simulink model "wr_model"  (R2018b)
settings: Solver=VariableStepAuto  StartTime=0.0  StopTime=20  FixedStep=1  MaxStep=10.0  RelTol=1e-3
undefined symbols (not defined in the file): water, wr
libraries: simulink x4
settings Model: Creator=martin  LastModifiedBy=felix
settings DataIOCC: OutputSaveName=State

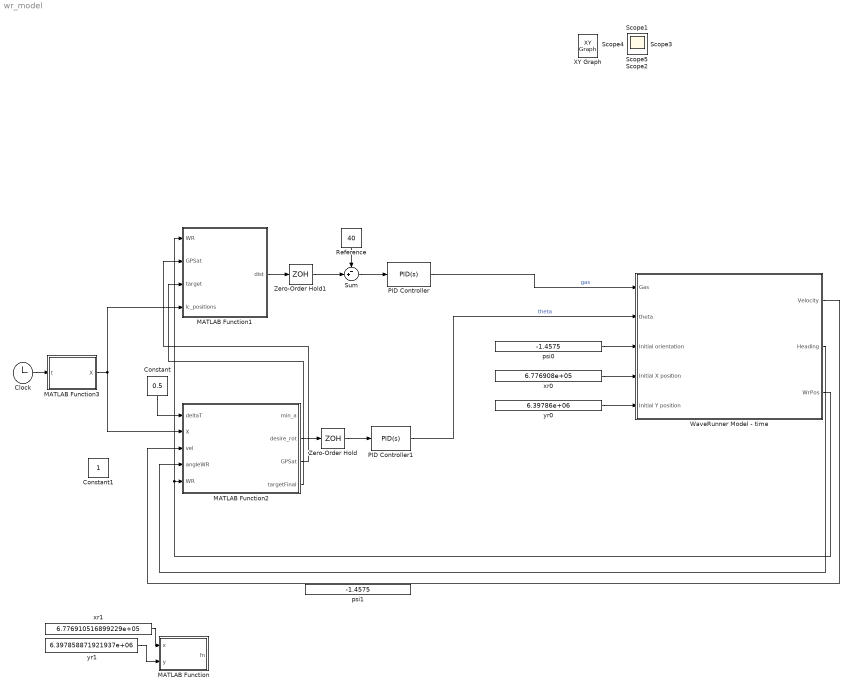
== system wr_model ==
  Clock : Clock
      settings: Decimation=1000
  Constant : Constant  Value=0.5
  Constant1 : Constant
  MATLAB Function : MATLAB Function  TreatAsAtomicUnit=on
  MATLAB Function1 : MATLAB Function  TreatAsAtomicUnit=on
  MATLAB Function2 : MATLAB Function  TreatAsAtomicUnit=on
  MATLAB Function3 : MATLAB Function  TreatAsAtomicUnit=on
  PID Controller : simulink/Continuous/PID Controller  Controller=PID  Form=Parallel  TimeDomain=Continuous-time  SampleTime=-1  IntegratorMethod=Forward Euler  FilterMethod=Forward Euler  ControllerParametersSource=internal  P=1  I=0  D=1  UseFilter=on  N=100  TunerSelectOption=Transfer Function Based (PID Tuner App)  InitialConditionSource=internal  InitialConditionForIntegrator=0  InitialConditionForFilter=0  DifferentiatorICPrevScaledInput=0  ExternalReset=none  TrackingMode=off  Kt=1  LimitOutput=on  UpperSaturationLimit=100  LowerSaturationLimit=0  LinearizeAsGain=off  AntiWindupMode=none  Kb=1  POutMin=[]  POutMax=[]  IOutMin=[]  IOutMax=[]  DOutMin=[]  DOutMax=[]  NOutMin=[]  NOutMax=[]  SumOutMin=[]  SumOutMax=[]  SaturationOutMin=[]  SaturationOutMax=[]  PParamMin=[]  PParamMax=[]  IParamMin=[]  IParamMax=[]  DParamMin=[]  DParamMax=[]  NParamMin=[]  NParamMax=[]  KbParamMin=[]  KbParamMax=[]  KtParamMin=[]  KtParamMax=[]  KbOutMin=[]  KbOutMax=[]  KtOutMin=[]  KtOutMax=[]  IntegratorOutMin=[]  IntegratorOutMax=[]  FilterOutMin=[]  FilterOutMax=[]  SumI1OutMin=[]  SumI1OutMax=[]  SumI2OutMin=[]  SumI2OutMax=[]  SumI3OutMin=[]  SumI3OutMax=[]  SumI4OutMin=[]  SumI4OutMax=[]  SumDOutMin=[]  SumDOutMax=[]  DifferentiatorOutMin=[]  DifferentiatorOutMax=[]  FilterDiffOutCoefMin=[]  FilterDiffOutCoefMax=[]  ReciprocalOutMin=[]  ReciprocalOutMax=[]  SumDenOutMin=[]  SumDenOutMax=[]  SumNumOutMin=[]  SumNumOutMax=[]  DivideOutMin=[]  DivideOutMax=[]  IntegratorContinuousStateAttributes=''  IntegratorStateMustResolveToSignalObject=off  IntegratorRTWStateStorageClass=Auto  FilterContinuousStateAttributes=''  FilterStateMustResolveToSignalObject=off  FilterRTWStateStorageClass=Auto  ParallelPVariant=InternalParameters  IdealPVariant=Disabled  IVariant=InternalParameters  DVariant=InternalParameters  IntegratorVariant=Continuous  SatVariant=Enabled  AWVariant=Passthrough  PCopyVariant=Disabled  TRVariant=Disabled  FdbkBlocksVariant=Forward  IdealPFdbkVariant=Disabled  SatFdbkVariant=Disabled  DerivativeFilterVariant=ContFilter  NVariant=InternalParameters  NCopyVariant=Disabled  FilterICVariant=InternalICsFilter  IntegratorICVariant=InternalICs  ExternalResetVariant=Disabled  TRSumVariant=Passthrough  SumFdbkVariant=Disabled  SumVariant=Sum_PID
  PID Controller1 : simulink/Continuous/PID Controller  Controller=PID  Form=Parallel  TimeDomain=Continuous-time  SampleTime=-1  IntegratorMethod=Forward Euler  FilterMethod=Forward Euler  ControllerParametersSource=internal  P=1  I=0  D=0  UseFilter=on  N=100  TunerSelectOption=Transfer Function Based (PID Tuner App)  InitialConditionSource=internal  InitialConditionForIntegrator=0  InitialConditionForFilter=0  DifferentiatorICPrevScaledInput=0  ExternalReset=none  TrackingMode=off  Kt=1  LimitOutput=on  UpperSaturationLimit=24*pi/180  LowerSaturationLimit=-24*pi/180  LinearizeAsGain=off  AntiWindupMode=none  Kb=1  POutMin=[]  POutMax=[]  IOutMin=[]  IOutMax=[]  DOutMin=[]  DOutMax=[]  NOutMin=[]  NOutMax=[]  SumOutMin=[]  SumOutMax=[]  SaturationOutMin=[]  SaturationOutMax=[]  PParamMin=[]  PParamMax=[]  IParamMin=[]  IParamMax=[]  DParamMin=[]  DParamMax=[]  NParamMin=[]  NParamMax=[]  KbParamMin=[]  KbParamMax=[]  KtParamMin=[]  KtParamMax=[]  KbOutMin=[]  KbOutMax=[]  KtOutMin=[]  KtOutMax=[]  IntegratorOutMin=[]  IntegratorOutMax=[]  FilterOutMin=[]  FilterOutMax=[]  SumI1OutMin=[]  SumI1OutMax=[]  SumI2OutMin=[]  SumI2OutMax=[]  SumI3OutMin=[]  SumI3OutMax=[]  SumI4OutMin=[]  SumI4OutMax=[]  SumDOutMin=[]  SumDOutMax=[]  DifferentiatorOutMin=[]  DifferentiatorOutMax=[]  FilterDiffOutCoefMin=[]  FilterDiffOutCoefMax=[]  ReciprocalOutMin=[]  ReciprocalOutMax=[]  SumDenOutMin=[]  SumDenOutMax=[]  SumNumOutMin=[]  SumNumOutMax=[]  DivideOutMin=[]  DivideOutMax=[]  IntegratorContinuousStateAttributes=''  IntegratorStateMustResolveToSignalObject=off  IntegratorRTWStateStorageClass=Auto  FilterContinuousStateAttributes=''  FilterStateMustResolveToSignalObject=off  FilterRTWStateStorageClass=Auto  ParallelPVariant=InternalParameters  IdealPVariant=Disabled  IVariant=InternalParameters  DVariant=InternalParameters  IntegratorVariant=Continuous  SatVariant=Enabled  AWVariant=Passthrough  PCopyVariant=Disabled  TRVariant=Disabled  FdbkBlocksVariant=Forward  IdealPFdbkVariant=Disabled  SatFdbkVariant=Disabled  DerivativeFilterVariant=ContFilter  NVariant=InternalParameters  NCopyVariant=Disabled  FilterICVariant=InternalICsFilter  IntegratorICVariant=InternalICs  ExternalResetVariant=Disabled  TRSumVariant=Passthrough  SumFdbkVariant=Disabled  SumVariant=Sum_PID
  Reference : Constant  Value=40
  Sum : Sum  Inputs=-+|
  WaveRunner Model - time : Subsystem
  Zero-Order Hold : ZeroOrderHold
  Zero-Order Hold1 : ZeroOrderHold
  psi0 : Constant  Value=-1.4575
  psi1 : Constant  Value=-1.4575
  xr0 : Constant  Value=6.776908e+05
  xr1 : Constant  Value=6.776910516899229e+05
  yr0 : Constant  Value=6.39786e+06
  yr1 : Constant  Value=6.397858871921937e+06
  Scope{,1..5} (6 alike) : Scope
  XY Graph : simulink/Sinks/XY Graph  IOType=viewer  xmin=-1  xmax=1  ymin=-1  ymax=1  st=-1
  wires:
  Clock/1 -> MATLAB Function3/1(t)
  MATLAB Function3/1(X) -> MATLAB Function1/4(lc_positions), MATLAB Function2/2(X)
  Constant/1 -> MATLAB Function2/1(deltaT)
  Reference/1 -> Sum/1
  MATLAB Function1/1(dist) -> Zero-Order Hold1/1
  psi0/1 -> WaveRunner Model - time/3(Initial orientation)
  xr0/1 -> WaveRunner Model - time/4(Initial X position)
  yr0/1 -> WaveRunner Model - time/5(Initial Y position)
  MATLAB Function2/3(GPSat) -> MATLAB Function1/2(GPSat)
  MATLAB Function2/4(targetFinal) -> MATLAB Function1/3(target)
  xr1/1 -> MATLAB Function/1(x)
  yr1/1 -> MATLAB Function/2(y)
  WaveRunner Model - time/3(WrPos) -> MATLAB Function1/1(WR), MATLAB Function2/5(WR)
  Zero-Order Hold/1 -> PID Controller1/1
  MATLAB Function2/2(desire_rot) -> Zero-Order Hold/1
  Zero-Order Hold1/1 -> Sum/2
  WaveRunner Model - time/2(Heading) -> MATLAB Function2/4(angleWR)
  WaveRunner Model - time/1(Velocity) -> MATLAB Function2/3(vel)
  Sum/1 -> PID Controller/1
  PID Controller/1 -> WaveRunner Model - time/1(Gas)  "gas"
  PID Controller1/1 -> WaveRunner Model - time/2(theta)  "theta"

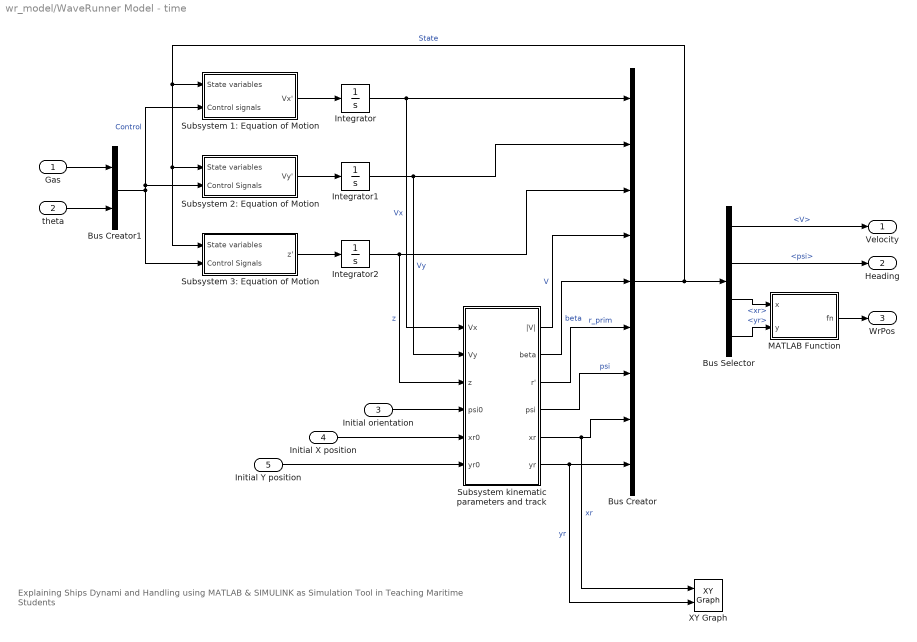
== system wr_model/WaveRunner Model - time ==
  note: Explaining Ships Dynami and Handling using MATLAB & SIMULINK as Simulation Tool in Teaching Maritime Students
  Gas : Inport
  theta : Inport  Port=2
  Initial orientation : Inport  Port=3
  Initial X position : Inport  Port=4
  Initial Y position : Inport  Port=5
  Bus Creator : BusCreator  Inputs=9
  Bus Creator1 : BusCreator  Inputs=2
  Bus Selector : BusSelector  OutputSignals=V,psi,xr,yr
  Integrator : Integrator
  Integrator1 : Integrator
  Integrator2 : Integrator
  MATLAB Function : MATLAB Function  TreatAsAtomicUnit=on
  Subsystem 1: Equation of Motion : Subsystem
  Subsystem 2: Equation of Motion : Subsystem
  Subsystem 3: Equation of Motion : Subsystem
  Subsystem kinematic parameters and track : Subsystem
  XY Graph : simulink/Sinks/XY Graph  xmin=6.65510516899229e+05  xmax=6.796910516899229e+05  ymin=6.308058871921937e+06  ymax=6.417858871921937e+06  st=-1
  Velocity : Outport
  Heading : Outport  Port=2
  WrPos : Outport  Port=3
  wires:
  Initial X position/1 -> Subsystem kinematic parameters and track/5(xr0)
  Subsystem 2: Equation of Motion/1(Vy') -> Integrator1/1
  Bus Creator/1 -> Subsystem 3: Equation of Motion/1(State variables), Subsystem 2: Equation of Motion/1(State variables), Subsystem 1: Equation of Motion/1(State variables), Bus Selector/1  "State"
  Integrator2/1 -> Subsystem kinematic parameters and track/3(z), Bus Creator/3  "z"
  Initial orientation/1 -> Subsystem kinematic parameters and track/4(psi0)
  Subsystem kinematic parameters and track/3(r') -> Bus Creator/6  "r_prim"
  Subsystem 1: Equation of Motion/1(Vx') -> Integrator/1
  Subsystem kinematic parameters and track/5(xr) -> XY Graph/1, Bus Creator/8  "xr"
  Subsystem kinematic parameters and track/6(yr) -> XY Graph/2, Bus Creator/9  "yr"
  Subsystem kinematic parameters and track/2(beta) -> Bus Creator/5  "beta"
  Bus Creator1/1 -> Subsystem 1: Equation of Motion/2(Control signals), Subsystem 2: Equation of Motion/2(Control Signals), Subsystem 3: Equation of Motion/2(Control Signals)  "Control"
  Subsystem kinematic parameters and track/4(psi) -> Bus Creator/7  "psi"
  Gas/1 -> Bus Creator1/1
  Integrator1/1 -> Subsystem kinematic parameters and track/2(Vy), Bus Creator/2  "Vy"
  Initial Y position/1 -> Subsystem kinematic parameters and track/6(yr0)
  Subsystem 3: Equation of Motion/1(z') -> Integrator2/1
  Subsystem kinematic parameters and track/1(|V|) -> Bus Creator/4  "V"
  Integrator/1 -> Bus Creator/1, Subsystem kinematic parameters and track/1(Vx)  "Vx"
  Bus Selector/2 -> Heading/1  "<psi>"
  Bus Selector/1 -> Velocity/1  "<V>"
  MATLAB Function/1(fn) -> WrPos/1
  theta/1 -> Bus Creator1/2
  Bus Selector/3 -> MATLAB Function/1(x)  "<xr>"
  Bus Selector/4 -> MATLAB Function/2(y)  "<yr>"

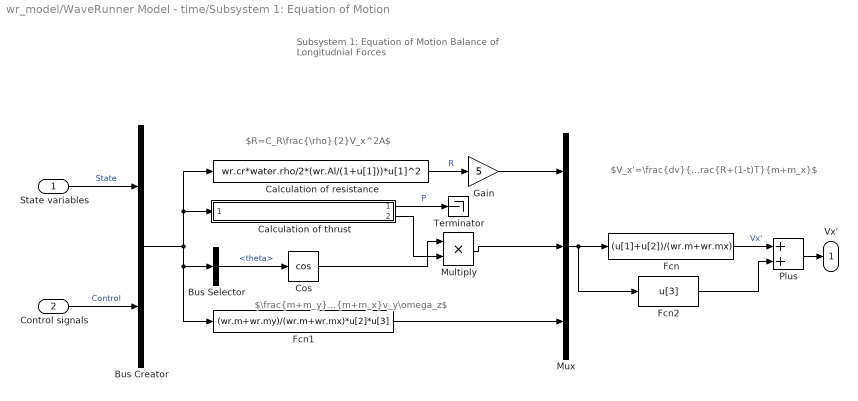
== system wr_model/WaveRunner Model - time/Subsystem 1: Equation of Motion ==
  note: $\frac{m+m_y}{m+m_x}v_y\omega_z$
  note: Subsystem 1: Equation of Motion
      | Balance of Longitudnial Forces
  note: $V_x'=\frac{dv}{dt}=\frac{R+(1-t)T}{m+m_x}$
  note: $R=C_R\frac{\rho}{2}V_x^2A$
  State variables : Inport
  Control signals : Inport  Port=2
  Bus Creator : BusCreator  Inputs=2  OutDataTypeStr=Bus: slBus1
  Bus Selector : BusSelector  OutputSignals=Control.theta
  Calculation of resistance : Fcn  Expr=wr.cr*water.rho/2*(wr.Al/(1+u[1]))*u[1]^2
  Calculation of thrust : ModelReference  ModelNameDialog=calculation_of_thrust  SimulationMode=Normal  ModelReferenceVersion=1.28
  Cos : Trigonometry  Operator=cos
  Fcn : Fcn  Expr=(u[1]+u[2])/(wr.m+wr.mx)
  Fcn1 : Fcn  Expr=(wr.m+wr.my)/(wr.m+wr.mx)*u[2]*u[3]
  Fcn2 : Fcn  Expr=u[3]
  Gain : Gain  Gain=5
  Multiply : Product
  Mux : Mux  Inputs=3
  Plus : Sum
  Terminator : Terminator
  Vx' : Outport
  wires:
  Mux/1 -> Fcn2/1, Fcn/1
  Calculation of resistance/1 -> Gain/1  "R"
  Control signals/1 -> Bus Creator/2  "Control"
  State variables/1 -> Bus Creator/1  "State"
  Plus/1 -> Vx'/1
  Bus Selector/1 -> Cos/1  "<theta>"
  Cos/1 -> Multiply/1
  Fcn1/1 -> Mux/3
  Bus Creator/1 -> Fcn1/1, Bus Selector/1, Calculation of resistance/1, Calculation of thrust/1
  Fcn/1 -> Plus/1  "Vx'"
  Fcn2/1 -> Plus/2
  Multiply/1 -> Mux/2
  Calculation of thrust/1 -> Terminator/1  "P"
  Gain/1 -> Mux/1
  Calculation of thrust/2 -> Multiply/2

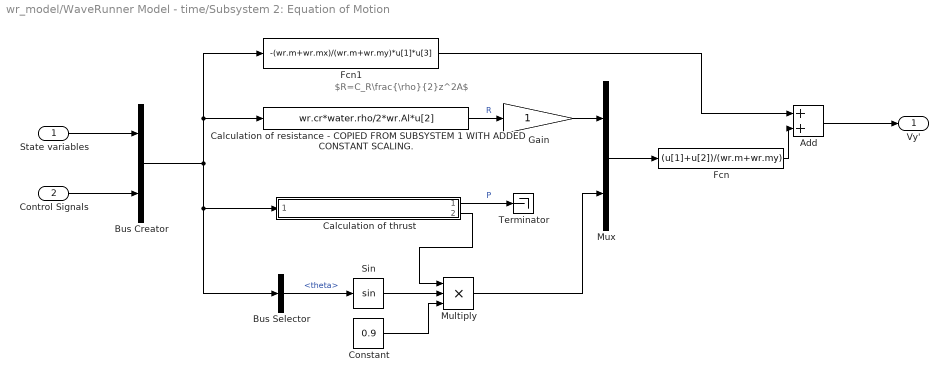
== system wr_model/WaveRunner Model - time/Subsystem 2: Equation of Motion ==
  note: $R=C_R\frac{\rho}{2}z^2A$
  State variables : Inport
  Control Signals : Inport  Port=2
  Add : Sum
  Bus Creator : BusCreator  Inputs=2
  Bus Selector : BusSelector  OutputSignals=Control.theta
  Calculation of resistance - COPIED FROM SUBSYSTEM 1 WITH ADDED CONSTANT SCALING. : Fcn  Expr=wr.cr*water.rho/2*wr.Al*u[2]
  Calculation of thrust : ModelReference  ModelNameDialog=calculation_of_thrust  SimulationMode=Normal  ModelReferenceVersion=1.28
  Constant : Constant  Value=0.9
  Fcn : Fcn  Expr=(u[1]+u[2])/(wr.m+wr.my)
  Fcn1 : Fcn  Expr=-(wr.m+wr.mx)/(wr.m+wr.my)*u[1]*u[3]
  Gain : Gain
  Multiply : Product  Inputs=3
  Mux : Mux  Inputs=2
  Sin : Trigonometry
  Terminator : Terminator
  Vy' : Outport
  wires:
  State variables/1 -> Bus Creator/1
  Control Signals/1 -> Bus Creator/2
  Calculation of resistance - COPIED FROM SUBSYSTEM 1 WITH ADDED CONSTANT SCALING./1 -> Gain/1  "R"
  Sin/1 -> Multiply/2
  Bus Selector/1 -> Sin/1  "<theta>"
  Constant/1 -> Multiply/3
  Bus Creator/1 -> Bus Selector/1, Calculation of thrust/1, Fcn1/1, Calculation of resistance - COPIED FROM SUBSYSTEM 1 WITH ADDED CONSTANT SCALING./1
  Mux/1 -> Fcn/1
  Gain/1 -> Mux/1
  Multiply/1 -> Mux/2
  Fcn/1 -> Add/2
  Fcn1/1 -> Add/1
  Add/1 -> Vy'/1
  Calculation of thrust/1 -> Terminator/1  "P"
  Calculation of thrust/2 -> Multiply/1

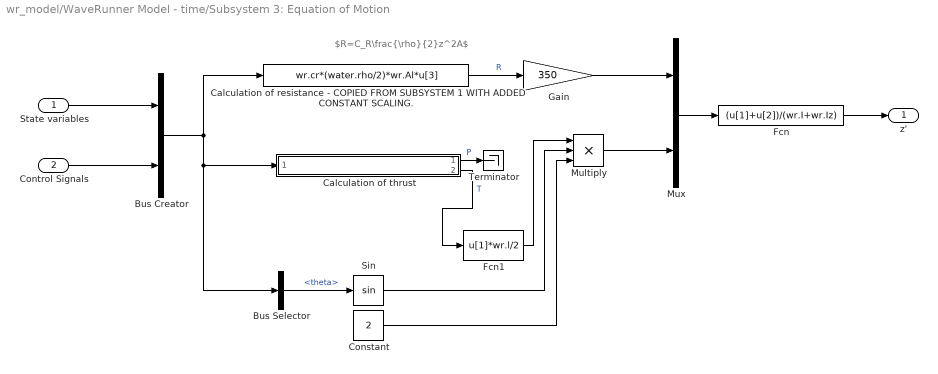
== system wr_model/WaveRunner Model - time/Subsystem 3: Equation of Motion ==
  note: $R=C_R\frac{\rho}{2}z^2A$
  State variables : Inport
  Control Signals : Inport  Port=2
  Bus Creator : BusCreator  Inputs=2
  Bus Selector : BusSelector  OutputSignals=Control.theta
  Calculation of resistance - COPIED FROM SUBSYSTEM 1 WITH ADDED CONSTANT SCALING. : Fcn  Expr=wr.cr*(water.rho/2)*wr.Al*u[3]
  Calculation of thrust : ModelReference  ModelNameDialog=calculation_of_thrust  SimulationMode=Normal  ModelReferenceVersion=1.28
  Constant : Constant  Value=2
  Fcn : Fcn  Expr=(u[1]+u[2])/(wr.I+wr.Iz)
  Fcn1 : Fcn  Expr=u[1]*wr.l/2
  Gain : Gain  Gain=350
  Multiply : Product  Inputs=3
  Mux : Mux  Inputs=2
  Sin : Trigonometry
  Terminator : Terminator
  z' : Outport
  wires:
  Control Signals/1 -> Bus Creator/2
  State variables/1 -> Bus Creator/1
  Sin/1 -> Multiply/2
  Bus Selector/1 -> Sin/1  "<theta>"
  Bus Creator/1 -> Calculation of resistance - COPIED FROM SUBSYSTEM 1 WITH ADDED CONSTANT SCALING./1, Bus Selector/1, Calculation of thrust/1
  Calculation of resistance - COPIED FROM SUBSYSTEM 1 WITH ADDED CONSTANT SCALING./1 -> Gain/1  "R"
  Multiply/1 -> Mux/2
  Fcn/1 -> z'/1
  Mux/1 -> Fcn/1
  Gain/1 -> Mux/1
  Fcn1/1 -> Multiply/1
  Calculation of thrust/2 -> Fcn1/1  "T"
  Calculation of thrust/1 -> Terminator/1  "P"
  Constant/1 -> Multiply/3

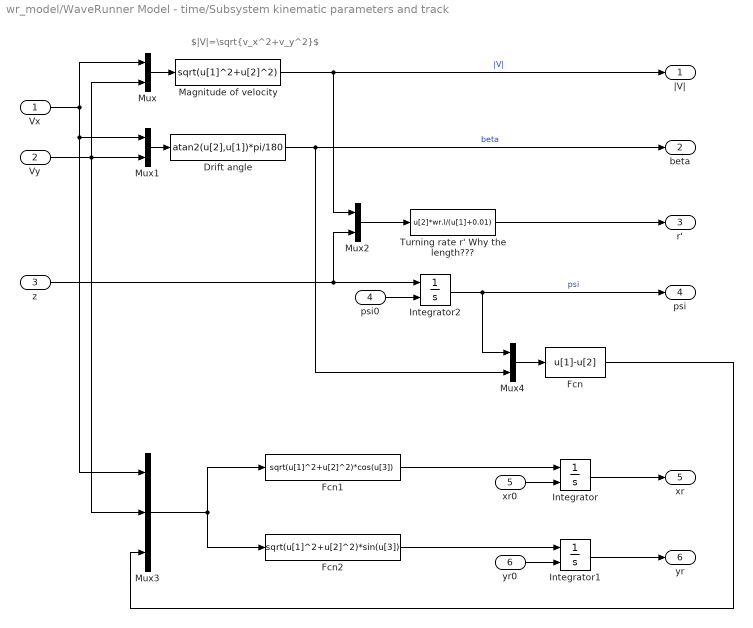
== system wr_model/WaveRunner Model - time/Subsystem kinematic parameters and track ==
  note: $|V|=\sqrt{v_x^2+v_y^2}$
  Vx : Inport
  Vy : Inport  Port=2
  z : Inport  Port=3
  psi0 : Inport  Port=4
  xr0 : Inport  Port=5
  yr0 : Inport  Port=6
  Drift angle : Fcn  Expr=atan2(u[2],u[1])*pi/180
  Fcn : Fcn  Expr=u[1]-u[2]
  Fcn1 : Fcn  Expr=sqrt(u[1]^2+u[2]^2)*cos(u[3])
  Fcn2 : Fcn  Expr=sqrt(u[1]^2+u[2]^2)*sin(u[3])
  Integrator : Integrator  InitialConditionSource=external
  Integrator1 : Integrator  InitialConditionSource=external
  Integrator2 : Integrator  InitialConditionSource=external
  Magnitude of velocity : Fcn  Expr=sqrt(u[1]^2+u[2]^2)
  Mux{,1..2,4} (4 alike) : Mux  Inputs=2
  Mux3 : Mux  Inputs=3
  Turning rate r' Why the length??? : Fcn  Expr=u[2]*wr.l/(u[1]+0.01)
  |V| : Outport
  beta : Outport  Port=2
  r' : Outport  Port=3
  psi : Outport  Port=4
  xr : Outport  Port=5
  yr : Outport  Port=6
  wires:
  Mux/1 -> Magnitude of velocity/1
  Magnitude of velocity/1 -> Mux2/1, |V|/1  "|V|"
  Vx/1 -> Mux/1, Mux3/1, Mux1/1
  Vy/1 -> Mux/2, Mux3/2, Mux1/2
  Integrator1/1 -> yr/1
  Integrator/1 -> xr/1
  Integrator2/1 -> Mux4/1, psi/1  "psi"
  psi0/1 -> Integrator2/2
  xr0/1 -> Integrator/2
  yr0/1 -> Integrator1/2
  z/1 -> Mux2/2, Integrator2/1
  Mux1/1 -> Drift angle/1
  Drift angle/1 -> Mux4/2, beta/1  "beta"
  Mux2/1 -> Turning rate r' Why the length???/1
  Turning rate r' Why the length???/1 -> r'/1
  Mux4/1 -> Fcn/1
  Fcn/1 -> Mux3/3
  Fcn1/1 -> Integrator/1
  Fcn2/1 -> Integrator1/1
  Mux3/1 -> Fcn1/1, Fcn2/1

== matlab function wr_model/MATLAB Function1 ==
  data: WR input; GPSat input; target input; lc_positions input; dist output
function dist  = distance_to_lc(WR, GPSat, target, lc_positions)
A = [lc_positions(1,GPSat+1), lc_positions(2,GPSat+1)];
%A = lc_positions(:,GPSat+1);
TargetToNext = norm(A - target);
DistToTarget = norm(target - WR);
dist = DistToTarget + TargetToNext;
for i = GPSat+1:length(lc_positions)-1
    %A = lc_positions(:,i);     
    A = [lc_positions(1,i), lc_positions(2,i)];
    %B = lc_positions(:,i+1);   
    B = [lc_positions(1,i+1), lc_positions(2,i+1)];
    C = B-A;
    dist = dist + norm(C);
end

== matlab function wr_model/WaveRunner Model - time/MATLAB Function ==
  data: x input; fn output; y input
function fn = fcn(x,y)
fn = [x, y];

== matlab function wr_model/MATLAB Function2 ==
  data: deltaT input; X input; vel input; min_a output; angleWR input; WR input; desire_rot output; GPSat output; targetFinal output
function [min_a, desire_rot, GPSat, targetFinal] =  rotation_of_wr_3(deltaT, X, vel,angleWR, WR)
% Description: 
% Calculates the rotation needed from the WR to reach the path (X) using
% a look-ahead method.
%
% Inputs:
% vel = velocity of the WR.
% deltaT = time intervall.
% dir_start = the current direction of the WR as a vector. 
% X = the matrix with all the path points.
% WR = current position of the WaveRunner.
%
% Outputs:
% min_a = the shortest distance found to the path from the WR.
% desire_rot = rotation difference between dir_start to the goal direction.
%
NotUsed = 0;
desire_rot = 0;
A = zeros(1,2);
B = zeros(1,2);
j = 0;
dir_start = [cos(angleWR),sin(angleWR)];
if vel ~= 0
    vel_vector = vel*deltaT*(dir_start/norm(dir_start));
else
    vel_vector = 0.2*dir_start/norm(dir_start);
end
predictLoc = WR + vel_vector;

min_a = 10^100;
% Loop through the X matrix (our path) to see which points the WR are
% closest to at this moment.
for i = 1:size(X,2)-1
    % Calculating howFar on current distance, distance to path.
    [NotUsed, howFar, NotUsed, a, NotUsed, NotUsed, NotUsed] = distance_to_path([X(1,i),X(2,i)],[X(1,i+1),X(2,i+1)],predictLoc);
%    [NotUsed, howFar, v, a, NotUsed, b, NotUsed] = distance_to_path(X(:,i), X(:,1+1), predictLoc);
    
    if (howFar < 1 && howFar > 0) 
        % Save the closest points to the WR on the path.     
        if (norm(a) < min_a)
            min_a = norm(a);
            
            A = [X(1,i), X(2,i)];
            B = [X(1,i+1), X(2,i+1)];
            j = i;
            break;
        end
    end
end

% Calculating distance to path and distance b = distance A -> predictLoc
[NotUsed, NotUsed, v, a, NotUsed, b, NotUsed] = distance_to_path(A,B,predictLoc);

% First target point calculated with our current speed and time interval +
% the current point + the "b" distance. 
target = (A+b) + vel.*deltaT.*(v/norm(v));

% Calculate howFar and distance c = distance B -> target
[NotUsed, howFar_target, NotUsed, NotUsed, NotUsed, NotUsed, dist_c_target] = distance_to_path(A,B,target);

% While the target point is to far ahead from our current PathPoints
% keep updating the distance left.
while(howFar_target > 1)
    AA = [X(1,j+1), X(2,j+1)];
    BB = [X(1,j+2), X(2,j+2)];
    j = j+1;
    s = abs(dist_c_target);
    
    [NotUsed, howFar_target, v_target, NotUsed, NotUsed, NotUsed, dist_c_target] = distance_to_path(AA,BB,target);
    % The target point using our last point plus the remaining distance
    % from our last target in the direction of the new line between AA and
    % BB
    target = AA + s*(v_target/norm(v_target));
end

% Calculate the rotation difference needed to reach the targetlocation
% from our current direction.
wr_to_target = target-WR;
targetFinal = target;
GPSat = j;
deg_WR = atan2(vel_vector(2), vel_vector(1));
% (Unused atm)   deg_Path = atand(v(2)/v(1));
deg_wr_to_target = atan2(wr_to_target(2), wr_to_target(1));
%change order here to flip Coordinate system 90Degrees anticlockwise
desire_rot = deg_WR - deg_wr_to_target;

== matlab function wr_model/MATLAB Function3 ==
  data: X output; t input
function X  = fcn(t)
if t > 5
    idx = floor(t) + 1;
else
    idx = 5;
end
a = 0;
coder.extrinsic('fscanf')
fileID = fopen('test1.txt','r');                            %S?g vilken fil och att vi vill l?sa
sizeX = [2, idx];
Y = zeros(2,idx);
X = zeros(2, 100);                                                      %orleken p? matrisen vi ska f? ut
formatSpec = '%f';                                          %Ange formatet som talen ska l?sas i (float)
[Y, count] = fscanf(fileID,formatSpec,sizeX);
for i = 1:length(Y)
    X(1,i) = Y(1,i);
    X(2,i) = Y(2,i);
end
a = size(X,2);                                              %Ge oss matrisen X l?st ifr?n filen, returnar ?ven antalet tal i filen.
for  i = 1:100 
     if i <= idx                                               %Loopa igenom matrisen och                                                         
        [X(1,i), X(2,i)] = deg2utm(X(1,i), X(2,i));
     else
         X(1,i) = X(1,idx);
         X(2,i) = X(2,idx);
     end                                                          %g?r om varje koordinat till
end

== matlab function wr_model/MATLAB Function ==
  data: x input; fn output; y input
function fn = fcn(x,y)
fn = [x, y];
